simulink model "ThreePhaseVectorControl"  (R2020a)
settings: Solver=ode15s  StartTime=0.0  StopTime=2.5  MaxStep=1e-6  RelTol=1e-6
model workspace (MAT data in the model file):
  frequency = 1
values from neighbouring files (symbols this model uses):
  Buffer = 500    [PLLFYP.m]
  Ki_PLL = 0.005    [PLLFYP.m]
  Kp_PLL = 0.05    [PLLFYP.m]
  Kp_VSC = 500    [PLLFYP.m]
  Lf = 0.005    [PLLFYP.m]
  Lg = XR*Rg/(100*pi)    [PLLFYP.m]
  MPM_Ts = 1/5000    (= 0.0002)    [PLLFYP.m]
  Rf = 0.1    [PLLFYP.m]
  Rg = sqrt((1/(1+XR^2))*((500^2)/(Pn*SCR))^2)    [PLLFYP.m]
  Vdc = 2000    [PLLFYP.m]
  wL = 2*pi*50*Lf    (= 1.57079632679)    [PLLFYP.m]
  wn = 3000    [PLLFYP.m]
  zeta = 0.707    [PLLFYP.m]
undefined symbols (not defined in the file or in its folder): Ki_PQ, Kp_PQ, mpm_wc, plecs, Q, Q_KF, R, wb, wc, wc1, wc2
libraries: powerlib_meascontrol x57, powerlib x25, simulink x4, eeStairGenerator x4, powerlib_extras x2, cstblocks x2
(part 1 of 4)
settings Model: SimulationMode=accelerator  Creator=behroozb  LastModifiedBy=aaron
settings SolverCC: MaxConsecutiveZCs=10000  ZeroCrossAlgorithm=Adaptive  AlgebraicLoopSolver=LineSearch
settings DataIOCC: ReturnWorkspaceOutputs=off
settings OptimizationCC: LifeSpan=inf
settings DebuggingCC: IgnoredZcDiagnostic=none  SFUnexpectedBacktrackingDiag=warning  SFNoUnconditionalDefaultTransitionDiag=warning  SFExecutionAtInitializationDiag=none  ArithmeticOperatorsInVariantConditions=warning
settings SFSimCC: SimUseLocalCustomCode=off  CustomCodeUndefinedFunction=UseInterfaceOnly
settings RTWCC: RTWUseLocalCustomCode=off
settings CodeAppCC: StateflowObjectComments=on
settings GRTTargetCC: TargetLangStandard=C89/C90 (ANSI)
settings ConfigComp: CovMetricSettings=dw  CovHtmlReporting=on  CovSaveCumulativeToWorkspaceVar=on  CovSaveSingleToWorkspaceVar=on  CovExternalEMLEnable=off
settings SimscapeCC: SimscapeNormalizeSystem=off

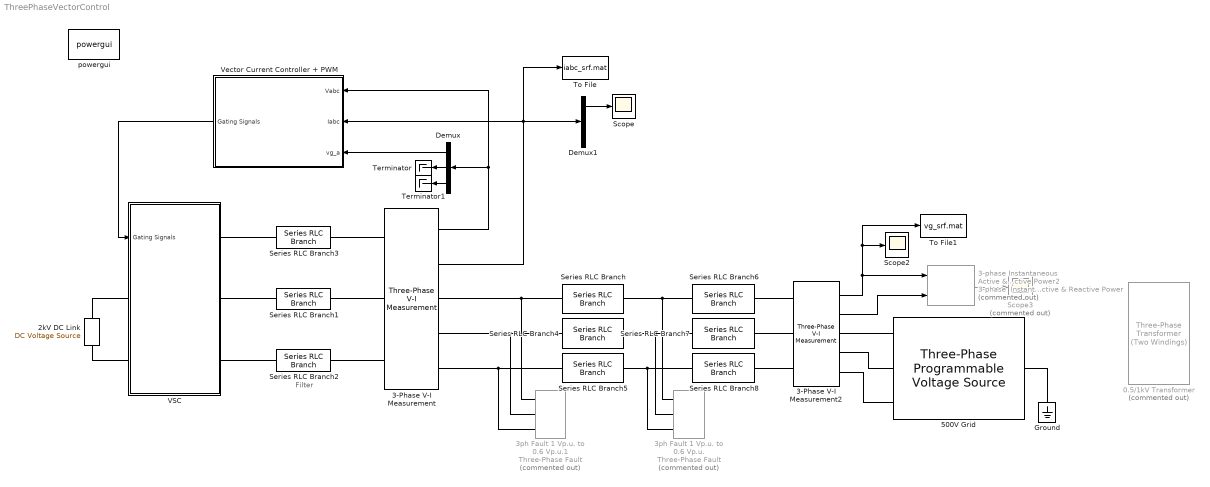
== system ThreePhaseVectorControl ==
  note: Filter
  0.5/1kV Transformer : powerlib/Elements/Three-Phase Transformer (Two Windings)  Commented=on  Winding1Connection=Yg  Winding2Connection=Yg  CoreType=Three single-phase transformers  SetSaturation=off  Hysteresis=off  DataFile='hysteresis'  SetInitialFlux=off  Measurements=None  UNITS=pu  NominalPower=[1e5 , 50]  Winding1=[500 , 0 , 0]  Winding2=[1000 , 0 , 0]  Rm=1e6  Lm=inf  L0=0.5  Saturation=[0 0;2.2531e-05 1065.2;0.0093878 1349.3]  InitialFluxes=[ 0.8 , -0.8 , 0.7 ]  BreakLoop=off  DiscreteSolver=Trapezoidal iterative  DataType=off  TransfoNumber=1
  2kV DC Link : powerlib/Electrical Sources/DC Voltage Source  Amplitude=Vdc  Measurements=None
  3-Phase V-I Measurement : powerlib/Measurements/Three-Phase V-I Measurement  VoltageMeasurement=phase-to-ground  SetLabelV=off  LabelV=Vabc  Vpu=off  VpuLL=off  CurrentMeasurement=yes  SetLabelI=off  LabelI=Iabc  Ipu=off  Pbase=100e6  Vbase=500e3  OutputType=Complex  PhasorSimulation=off  PSBequivalent=0
  3-Phase V-I Measurement2 : powerlib/Measurements/Three-Phase V-I Measurement  VoltageMeasurement=phase-to-ground  SetLabelV=off  LabelV=Vabc  Vpu=off  VpuLL=off  CurrentMeasurement=yes  SetLabelI=off  LabelI=Iabc  Ipu=off  Pbase=100e6  Vbase=500e3  OutputType=Complex  PhasorSimulation=off  PSBequivalent=0
  3-phase Instantaneous Active & Reactive Power2 : powerlib_extras/Measurements/3-phase  Instantaneous  Active & Reactive Power  Commented=on
      settings: SourceProductBaseCode=PS
  3ph Fault 1 Vp.u. to 0.6 Vp.u. : powerlib/Elements/Three-Phase Fault  Commented=on  InitialStates=0  FaultA=on  FaultB=on  FaultC=on  GroundFault=on  SwitchTimes=[0.35 0.43]  External=off  SwitchStatus=NaN  FaultResistance=9.2  GroundResistance=0.0001  SnubberResistance=inf  SnubberCapacitance=inf  Measurements=None
  3ph Fault 1 Vp.u. to 0.6 Vp.u.1 : powerlib/Elements/Three-Phase Fault  Commented=on  InitialStates=0  FaultA=on  FaultB=on  FaultC=on  GroundFault=on  SwitchTimes=[0.35 0.43]  External=off  SwitchStatus=NaN  FaultResistance=9.2  GroundResistance=0.0001  SnubberResistance=inf  SnubberCapacitance=inf  Measurements=None
  500V Grid : powerlib/Electrical Sources/Three-Phase Programmable Voltage Source  PositiveSequence=[500 0 50]  VariationEntity=None  VariationType=Step  VariationTypeAlt=Ramp  VariationStep=-0.1  VariationRate=-1  VariationMagnitude=0.1  VariationFrequency=1  VariationTiming=[0.4 0.5]  VariationPhaseA=off  Amplitudes=[1 0.8 1.2 1.0]  TimeValues=[0 0.1 0.15 0.2]  HarmonicGeneration=off  HarmonicA=[1 0.2 -25 2]  HarmonicB=[2 0.0 35 2]  Timing="[0.05  3]"  BusType=swing  Pref=0  Qref=0  Qmin=-inf  Qmax=inf
  Demux : Demux  Outputs=3
  Demux1 : Demux  Outputs=3
  Ground : powerlib/Elements/Ground  LConnTagsString=a
  Scope : Scope
  Scope2 : Scope
  Scope3 : Scope  Commented=on
  Series RLC Branch{,4..8} (6 alike) : powerlib/Elements/Series RLC Branch  LConnTagsString=__new0  RConnTagsString=__new0  BranchType=RL  Resistance=Rg/2  Inductance=Lg/2  SetiL0=off  InitialCurrent=0  Capacitance=1e-6  Setx0=off  InitialVoltage=0  Measurements=None
  Series RLC Branch1 : powerlib/Elements/Series RLC Branch  LConnTagsString=__new0  RConnTagsString=__new0  BranchType=RL  Resistance=Rf  Inductance=Lf  SetiL0=off  InitialCurrent=0  Capacitance=1.0  Setx0=off  InitialVoltage=0  Measurements=None
  Series RLC Branch2 : powerlib/Elements/Series RLC Branch  LConnTagsString=__new0  RConnTagsString=__new0  BranchType=RL  Resistance=Rf  Inductance=Lf  SetiL0=off  InitialCurrent=0  Capacitance=1.0  Setx0=off  InitialVoltage=0  Measurements=None
  Series RLC Branch3 : powerlib/Elements/Series RLC Branch  LConnTagsString=__new0  RConnTagsString=__new0  BranchType=RL  Resistance=Rf  Inductance=Lf  SetiL0=off  InitialCurrent=0  Capacitance=1.0  Setx0=off  InitialVoltage=0  Measurements=None
  Terminator : Terminator
  Terminator1 : Terminator
  To File : ToFile  Filename=iabc_srf.mat  SaveFormat=Timeseries
  To File1 : ToFile  Filename=vg_srf.mat  SaveFormat=Timeseries
  VSC : Subsystem
  Vector Current Controller + PWM : Subsystem
  powergui : powerlib/powergui  Priority=1  SimulationMode=Continuous  SampleTime=10e-6  frequency=60  Iterations=50  frequencyindice=50  Pbase=100e6  ErrMax=1e-4  UnitsV=kV  UnitsW=MW  buscounter=0  FunctionMessages=off  echomessages=off  EnableUseOfTLC=off  CurrentSourceSwitches=off  DisableSnubberDevices=off  DisableRonSwitches=off  DisableVfSwitches=off  DisplayEquations=off  AutomaticDiscreteSolvers=off  SolverType=Tustin/Backward Euler (TBE)  Interpol=off  ExternalGateDelay=off  methode=off  Ts=100  x0status=blocks  SPID=on  SwTol=0  HookPort=off  NonlinearTolerance=1e-4  nMaxIteration=100  ContinueOnMaxIteration=off  RestoreLinks=warning  ResistiveCurrentMeasurement=off  Frange=[0:2:500]  Ylog=off  Xlog=on  ShowGrid=off  save=off  variable=ZData  structure=ScopeData1  ZoomFFT=off  StartTime=0.4  cycles=20  DisplayStyle=1  fundamental=50  FreqAxis=off  MaxFrequency=150  frequencyindicesteady=1  RmsSteady=1  display=off
  wires:
  Vector Current Controller + PWM/1(Gating Signals) -> VSC/1(Gating Signals)
  3-Phase V-I Measurement/1 -> Vector Current Controller + PWM/1(Vabc), Demux/1
  Demux/1 -> Vector Current Controller + PWM/3(vg_a)
  Demux/2 -> Terminator/1
  Demux/3 -> Terminator1/1
  3-Phase V-I Measurement/2 -> Demux1/1, To File/1, Vector Current Controller + PWM/2(Iabc)
  Demux1/1 -> Scope/1
  3-Phase V-I Measurement2/2 -> 3-phase Instantaneous Active & Reactive Power2/2
  3-phase Instantaneous Active & Reactive Power2/1 -> Scope3/1
  3-Phase V-I Measurement2/1 -> 3-phase Instantaneous Active & Reactive Power2/1, To File1/1, Scope2/1
  connections:
  2kV DC Link/RConn1 -- VSC/LConn1
  2kV DC Link/LConn1 -- VSC/LConn2
  Series RLC Branch3/LConn1 -- VSC/RConn1
  Series RLC Branch1/LConn1 -- VSC/RConn2
  Series RLC Branch2/LConn1 -- VSC/RConn3
  500V Grid/LConn1 -- Ground/LConn1
  3-Phase V-I Measurement/LConn1 -- Series RLC Branch3/RConn1
  3-Phase V-I Measurement/LConn2 -- Series RLC Branch1/RConn1
  Series RLC Branch2/RConn1 -- 3-Phase V-I Measurement/LConn3
  Series RLC Branch6/LConn1 -- 3ph Fault 1 Vp.u. to 0.6 Vp.u./LConn1 -- Series RLC Branch/RConn1
  Series RLC Branch7/LConn1 -- 3ph Fault 1 Vp.u. to 0.6 Vp.u./LConn2 -- Series RLC Branch4/RConn1
  Series RLC Branch8/LConn1 -- 3ph Fault 1 Vp.u. to 0.6 Vp.u./LConn3 -- Series RLC Branch5/RConn1
  3-Phase V-I Measurement2/LConn1 -- Series RLC Branch6/RConn1
  3-Phase V-I Measurement2/LConn2 -- Series RLC Branch7/RConn1
  3-Phase V-I Measurement2/LConn3 -- Series RLC Branch8/RConn1
  3-Phase V-I Measurement2/RConn1 -- 500V Grid/RConn1
  3-Phase V-I Measurement2/RConn2 -- 500V Grid/RConn2
  3-Phase V-I Measurement2/RConn3 -- 500V Grid/RConn3
  3-Phase V-I Measurement/RConn1 -- 3ph Fault 1 Vp.u. to 0.6 Vp.u.1/LConn1 -- Series RLC Branch/LConn1
  Series RLC Branch4/LConn1 -- 3ph Fault 1 Vp.u. to 0.6 Vp.u.1/LConn2 -- 3-Phase V-I Measurement/RConn2
  3-Phase V-I Measurement/RConn3 -- 3ph Fault 1 Vp.u. to 0.6 Vp.u.1/LConn3 -- Series RLC Branch5/LConn1

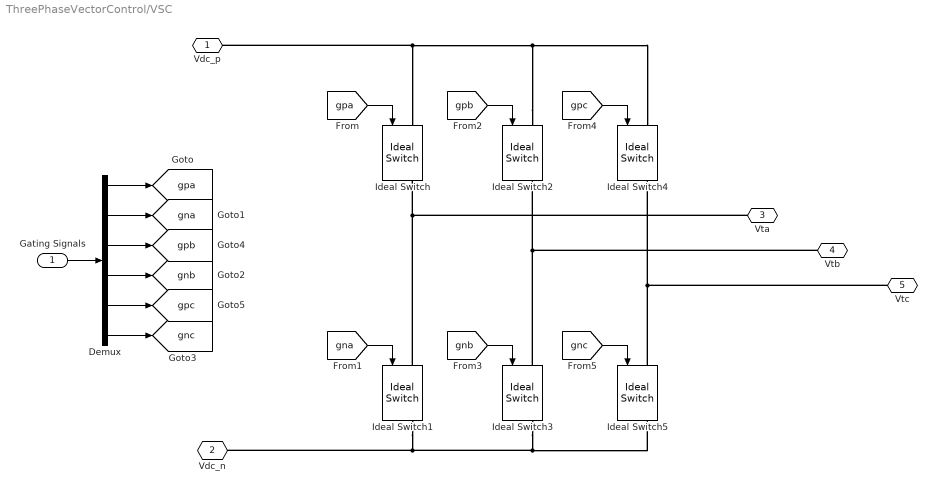
== system ThreePhaseVectorControl/VSC ==
  Gating Signals : Inport
  Demux : Demux  Outputs=6
  Ideal Switch{,1..5} (6 alike) : powerlib/Power Electronics/Ideal Switch  Ron=1e-6  Lon=0  IC=0  Rs=1e6  Cs=inf  Measurements=on
  Vdc_p : PMIOPort  Side=Left
  Vdc_n : PMIOPort  Port=2  Side=Left
  Vta : PMIOPort  Port=3  Side=Right
  Vtb : PMIOPort  Port=4  Side=Right
  Vtc : PMIOPort  Port=5  Side=Right
  tag scope: gna=global, gnb=global, gnc=global, gpa=global, gpb=global, gpc=global
  wires:
  [gpa] -> Ideal Switch/1
  [gpb] -> Ideal Switch2/1
  [gpc] -> Ideal Switch4/1
  [gna] -> Ideal Switch1/1
  [gnb] -> Ideal Switch3/1
  [gnc] -> Ideal Switch5/1
  Demux/3 -> [gpb]
  Demux/2 -> [gna]
  Demux/1 -> [gpa]
  Demux/4 -> [gnb]
  Demux/5 -> [gpc]
  Demux/6 -> [gnc]
  Gating Signals/1 -> Demux/1
  connections:
  Ideal Switch5/LConn1 -- Ideal Switch4/RConn1 -- Vtc/RConn1
  Ideal Switch3/LConn1 -- Ideal Switch2/RConn1 -- Vtb/RConn1
  Ideal Switch3/RConn1 -- Ideal Switch1/RConn1 -- Vdc_n/RConn1 -- Ideal Switch5/RConn1
  Ideal Switch1/LConn1 -- Vta/RConn1 -- Ideal Switch/RConn1
  Ideal Switch2/LConn1 -- Vdc_p/RConn1 -- Ideal Switch/LConn1 -- Ideal Switch4/LConn1

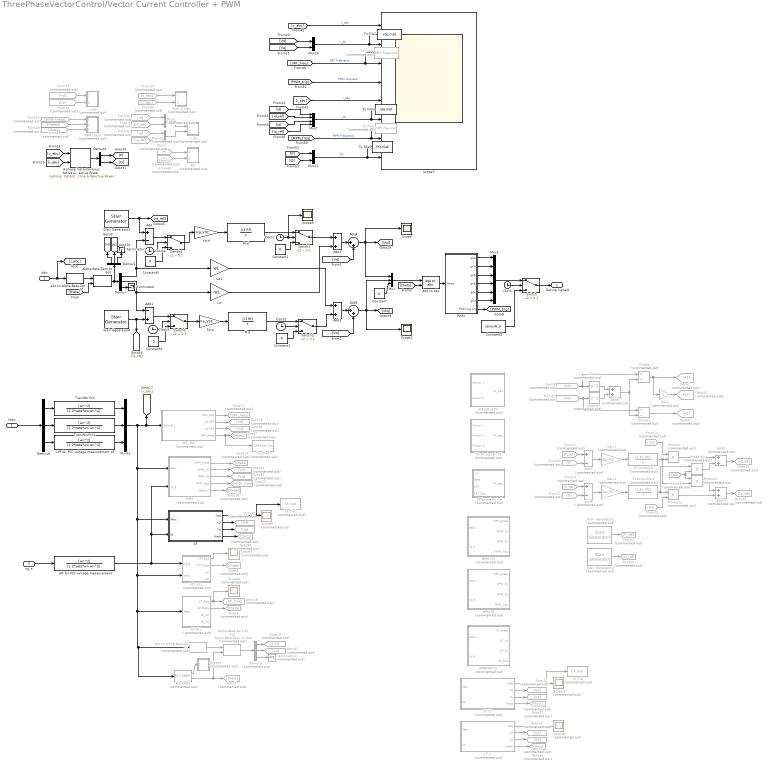
== system ThreePhaseVectorControl/Vector Current Controller + PWM ==
  Vabc : Inport
  Iabc : Inport  Port=2
  vg_a : Inport  Port=3
  3-phase Instantaneous Active & Reactive Power : powerlib_extras/Measurements/3-phase  Instantaneous  Active & Reactive Power
      settings: SourceProductBaseCode=PS
  Add : Sum  Inputs=+-
  Add1 : Sum  Inputs=-+
  Add10 : Sum  Commented=on
  Add2 : Sum
  Add3 : Sum
  Add4 : Sum  Inputs=|++
  Add5 : Sum  Inputs=|++
  Add6 : Sum  Commented=on
  Add7 : Sum  Commented=on  Inputs=+-
  Add8 : Sum  Commented=on  Inputs=+-
  Add9 : Sum  Commented=on
  Alpha-Beta-Zero to dq0 : powerlib_meascontrol/Transformations/Alpha-Beta-Zero to dq0  Alignment=Aligned with phase A axis
  Alpha-Beta-Zero to dq1 : powerlib_meascontrol/Transformations/Alpha-Beta-Zero to dq0  Commented=on  Alignment=Aligned with phase A axis
  CF : Subsystem
  CF (2) : Subsystem  Commented=on
  CF 2 : Subsystem  Commented=on
  CF based on i_d : Subsystem  Commented=on
  Clock{,1..4} (5 alike) : Clock
      settings: Decimation=100
  Constant{,1,3..5} (5 alike) : Constant  Value=0
  Constant2 : Constant  Value=zeros(6,1)
  Demux : Demux  Outputs=3
  Demux1 : Demux  Outputs=3
  Demux4 : Demux  Outputs=2
  Demux5 : Demux  Commented=on  Outputs=3
  Demux6 : Demux  Outputs=3
  Divide : Product  Commented=on  Inputs=*/
  Divide1 : Product  Commented=on  Inputs=*/
  FFT_PLL : Subsystem  Commented=on
  From10 : From  Commented=on  GotoTag=Vq
  From11 : From  Commented=on  GotoTag=P_ref
  From12 : From  Commented=on  GotoTag=Q
  From13 : From  Commented=on  GotoTag=Vd
  From14 : From  Commented=on  GotoTag=Vq
  From17 : From  Commented=on  GotoTag=MPM_theta
  From18 : From  Commented=on  GotoTag=theta0
  From19 : From  Commented=on  GotoTag=theta
  From22 : From  Commented=on  GotoTag=P
  From23 : From  Commented=on  GotoTag=Q_ref
  From24 : From  Commented=on  GotoTag=A1
  From25 : From  Commented=on  GotoTag=A3
  From26 : From  Commented=on  GotoTag=A2
  From34 : From  Commented=on  GotoTag=id
  From35 : From  Commented=on  GotoTag=iq
  From36 : From  Commented=on  GotoTag=i_abc
  From37 : From  Commented=on  GotoTag=v_abc
  From39 : From  Commented=on  GotoTag=P
  From40 : From  Commented=on  GotoTag=Q
  From7 : From  Commented=on  GotoTag=id_ref
  From8 : From  Commented=on  GotoTag=iq_ref
  From9 : From  Commented=on  GotoTag=Vd
  Gain : Gain  Commented=on  Gain=-1
  Gain1 : Gain  Commented=on  Gain=Kp_PQ
  Gain2 : Gain  Commented=on  Gain=Kp_PQ
  Goto1 : Goto  Commented=on  GotoTag=A1
  Goto11 : Goto  Commented=on  GotoTag=SRF_freq
  Goto12 : Goto  Commented=on  GotoTag=MPM_freq
  Goto{2,4..5,7,13,27,32,39} (8 alike) : Goto  Commented=on  GotoTag=theta
  Goto{14,19,25,33,35,37} (6 alike) : Goto  Commented=on  GotoTag=Vd
  Goto{15,26,34,36,38,47} (6 alike) : Goto  Commented=on  GotoTag=Vq
  Goto16 : Goto  Commented=on  GotoTag=KF_freq
  Goto18 : Goto  Commented=on  GotoTag=theta0
  Goto40 : Goto  Commented=on  GotoTag=A3
  Goto41 : Goto  Commented=on  GotoTag=id_ref
  Goto42 : Goto  Commented=on  GotoTag=iq_ref
  Goto43 : Goto  Commented=on  GotoTag=P_ref
  Goto44 : Goto  Commented=on  GotoTag=Q_ref
  Goto6 : Goto  Commented=on  GotoTag=A2
  KF_PLL : Subsystem  Commented=on
  Kp-d : Gain  Gain=Kp_VSC
  Kp-q : Gain  Gain=Kp_VSC
  LPF for PCC voltage measurement : TransferFcn  Numerator=[wn^2]  Denominator=[1 2*zeta*wn wn^2]
  LPF for PCC voltage measurement x3 : TransferFcn  Numerator=[wn^2]  Denominator=[1 2*zeta*wn wn^2]
  Lw : Gain  Gain=-wL
  Lw1 : Gain  Gain=wL
  MPM : Subsystem  Commented=on
  MPM CF : Subsystem  Commented=on
  MPM CF1 : Subsystem  Commented=on
  MPM theta : Subsystem  Commented=on  LoadFcn=plecs('sl', 300);  InitFcn=plecs('sl', 314);  StartFcn=plecs('sl', 308);  StopFcn=plecs('sl', 309);  mask{Settings=<binary blob, 1428 chars, not shown>}
      mask init:
      | plecs('sl', 315);
      settings: CopyFcn=plecs('sl', 303);  DeleteFcn=plecs('sl', 305);  UndoDeleteFcn=plecs('sl', 306);  PreSaveFcn=plecs('sl', 311);  NameChangeFcn=plecs('sl', 310);  DestroyFcn=plecs('sl', 307);  OpenFcn=plecs('sl', 302);  ErrorFcn=plerrorfcn
      mask Display: plot([0.1 0.9 0.9 0.1 0.1], [0.9 0.9 0.5 0.5 0.9])
  MPM/SRF CF : Subsystem  Commented=on
  Mux : Mux  Inputs=3
  Mux1 : Mux  Inputs=6
  Mux10 : Mux  Inputs=2
  Mux11 : Mux  Inputs=2
  Mux12 : Mux  Inputs=3
  Mux2 : Mux  Commented=on  Inputs=2
  Mux3 : Mux  Commented=on  Inputs=2
  Mux7 : Mux
  PI Controller : TransferFcn  Commented=on  Numerator=[1 Ki_PQ]  Denominator=[1 0]
  PI Controller1 : TransferFcn  Commented=on  Numerator=[1 Ki_PQ]  Denominator=[1 0]
  PI-d : TransferFcn  Numerator=[Lf Rf]  Denominator=[1 0]
  PI-q : TransferFcn  Numerator=[Lf Rf]  Denominator=[1 0]
  PLL (3ph) : powerlib_meascontrol/PLL/PLL (3ph)  Commented=on  Fmin=45  Par_Init=[0, 50]  ParK=[180, 3200, 1]  TcD=1e-4  MaxRateChangeFreq=12  FilterCutOffFreq=25  Ts=1e-4  AGC=on
  PQ : Subsystem  Commented=on  LoadFcn=plecs('sl', 300);  InitFcn=plecs('sl', 314);  StartFcn=plecs('sl', 308);  StopFcn=plecs('sl', 309);  mask{Settings=<binary blob, 1208 chars, not shown>}
      mask init:
      | plecs('sl', 315);
      settings: CopyFcn=plecs('sl', 303);  DeleteFcn=plecs('sl', 305);  UndoDeleteFcn=plecs('sl', 306);  PreSaveFcn=plecs('sl', 311);  NameChangeFcn=plecs('sl', 310);  DestroyFcn=plecs('sl', 307);  OpenFcn=plecs('sl', 302);  ErrorFcn=plerrorfcn
      mask Display: plot([0.1 0.9 0.9 0.1 0.1], [0.9 0.9 0.5 0.5 0.9])
  PWM : Subsystem
  Product{,1..3} (4 alike) : Product  Commented=on
  SRF_PLL : Subsystem  Commented=on
  Scope : Scope
  Scope1 : Subsystem  Commented=on  LoadFcn=plecs('sl', 300);  InitFcn=plecs('sl', 314);  StartFcn=plecs('sl', 308);  StopFcn=plecs('sl', 309);  mask{Settings=<binary blob, 1052 chars, not shown>}
      mask init:
      | plecs('sl', 315);
      settings: CopyFcn=plecs('sl', 303);  DeleteFcn=plecs('sl', 305);  UndoDeleteFcn=plecs('sl', 306);  PreSaveFcn=plecs('sl', 311);  NameChangeFcn=plecs('sl', 310);  DestroyFcn=plecs('sl', 307);  OpenFcn=plecs('sl', 302);  ErrorFcn=plerrorfcn
      mask Display: plot([0.1 0.9 0.9 0.1 0.1], [0.9 0.9 0.5 0.5 0.9])
  Scope2 : Scope
  Scope3 : Scope
  Scope{4..6,8..9} (5 alike) : Scope  Commented=on
  Scope7 : Scope  NumInputPorts=8
  Square : Math  Commented=on  Operator=square  SaturateOnIntegerOverflow=on
  Square1 : Math  Commented=on  Operator=square  SaturateOnIntegerOverflow=on
  Stair Generator1 : eeStairGenerator/Stair Generator  Commented=on  LabelModeActiveChoice=Discrete  TimeInput=[0 0.15]  AmplitudeInput=[0 1e4]  SampleTime=0.01  RepeatPattern=off  OutDataTypeStr=double
      settings: SourceProductBaseCode=PS
  Stair Generator2 : eeStairGenerator/Stair Generator  Commented=on  LabelModeActiveChoice=Discrete  TimeInput=[0]  AmplitudeInput=[0]  SampleTime=0.01  RepeatPattern=off  OutDataTypeStr=double
      settings: SourceProductBaseCode=PS
  Stair Generator3 : eeStairGenerator/Stair Generator  LabelModeActiveChoice=Discrete  TimeInput=[0 0.15]  AmplitudeInput=[0 50]  SampleTime=0.01  RepeatPattern=off  OutDataTypeStr=double
      settings: SourceProductBaseCode=PS
  Stair Generator4 : eeStairGenerator/Stair Generator  LabelModeActiveChoice=Discrete  TimeInput=[0]  AmplitudeInput=[0]  SampleTime=0.01  RepeatPattern=off  OutDataTypeStr=double
      settings: SourceProductBaseCode=PS
  Standard CF : Subsystem  Commented=on
  Switch{,1..4} (5 alike) : Switch  Criteria=u2 > Threshold  Threshold=0.1
  Terminator : Terminator
  Terminator1 : Terminator
  Terminator2 : Terminator  Commented=on
  Three signals CF : Subsystem  Commented=on
  To File : ToFile  Commented=on  Filename=CF.mat  SaveFormat=Timeseries
  To File1 : ToFile  Commented=on  Filename=CF.mat  SaveFormat=Timeseries
  To File2 : ToFile  Commented=on  Filename=MPM_freq.mat  SaveFormat=Timeseries
  To File3 : ToFile  Filename=idq.mat  SaveFormat=Timeseries
  To File4 : ToFile  Commented=on  Filename=SRF_freq.mat  SaveFormat=Timeseries
  To File5 : ToFile  Filename=PQ.mat  SaveFormat=Timeseries
  To File6 : ToFile  Commented=on  Filename=SRFtheta.mat  SaveFormat=Timeseries
  To File7 : ToFile  Filename=vdq.mat  SaveFormat=Timeseries
  Transfer Fcn : TransferFcn  Numerator=[wn^2]  Denominator=[1 2*zeta*wn wn^2]
  Transfer Fcn1 : TransferFcn  Numerator=[wn^2]  Denominator=[1 2*zeta*wn wn^2]
  Vabc & Iabc : Subsystem  Commented=on  LoadFcn=plecs('sl', 300);  InitFcn=plecs('sl', 314);  StartFcn=plecs('sl', 308);  StopFcn=plecs('sl', 309);  mask{Settings=<binary blob, 1272 chars, not shown>}
      mask init:
      | plecs('sl', 315);
      settings: CopyFcn=plecs('sl', 303);  DeleteFcn=plecs('sl', 305);  UndoDeleteFcn=plecs('sl', 306);  PreSaveFcn=plecs('sl', 311);  NameChangeFcn=plecs('sl', 310);  DestroyFcn=plecs('sl', 307);  OpenFcn=plecs('sl', 302);  ErrorFcn=plerrorfcn
      mask Display: plot([0.1 0.9 0.9 0.1 0.1], [0.9 0.9 0.5 0.5 0.9])
  abc to Alpha-Beta-Zero1 : powerlib_meascontrol/Transformations/abc to Alpha-Beta-Zero
  abc to Alpha-Beta-Zero2 : powerlib_meascontrol/Transformations/abc to Alpha-Beta-Zero  Commented=on
  dq0 to abc : powerlib_meascontrol/Transformations/dq0 to abc  Alignment=Aligned with phase A axis
  i_dq : Subsystem  Commented=on  LoadFcn=plecs('sl', 300);  InitFcn=plecs('sl', 314);  StartFcn=plecs('sl', 308);  StopFcn=plecs('sl', 309);  mask{Settings=<binary blob, 1256 chars, not shown>}
      mask init:
      | plecs('sl', 315);
      settings: CopyFcn=plecs('sl', 303);  DeleteFcn=plecs('sl', 305);  UndoDeleteFcn=plecs('sl', 306);  PreSaveFcn=plecs('sl', 311);  NameChangeFcn=plecs('sl', 310);  DestroyFcn=plecs('sl', 307);  OpenFcn=plecs('sl', 302);  ErrorFcn=plerrorfcn
      mask Display: plot([0.1 0.9 0.9 0.1 0.1], [0.9 0.9 0.5 0.5 0.9])
  v_dq : Subsystem  Commented=on  LoadFcn=plecs('sl', 300);  InitFcn=plecs('sl', 314);  StartFcn=plecs('sl', 308);  StopFcn=plecs('sl', 309);  mask{Settings=<binary blob, 1220 chars, not shown>}
      mask init:
      | plecs('sl', 315);
      settings: CopyFcn=plecs('sl', 303);  DeleteFcn=plecs('sl', 305);  UndoDeleteFcn=plecs('sl', 306);  PreSaveFcn=plecs('sl', 311);  NameChangeFcn=plecs('sl', 310);  DestroyFcn=plecs('sl', 307);  OpenFcn=plecs('sl', 302);  ErrorFcn=plerrorfcn
      mask Display: plot([0.1 0.9 0.9 0.1 0.1], [0.9 0.9 0.5 0.5 0.9])
  Gating Signals : Outport  VectorParamsAs1DForOutWhenUnconnected=off
  wires:
  Iabc/1 -> [i_abc], abc to Alpha-Beta-Zero1/1
  abc to Alpha-Beta-Zero1/1 -> Alpha-Beta-Zero to dq0/1
  [theta] -> Alpha-Beta-Zero to dq0/2
  Alpha-Beta-Zero to dq0/1 -> Demux1/1, Demux/1
  Demux/2 -> Lw/1, Add1/1
  Demux/1 -> Add/2, Lw1/1
  Add2/1 -> Add4/1
  Add3/1 -> Add5/1
  [theta] -> dq0 to abc/2
  dq0 to abc/1 -> PWM/1(Vtabc)
  Constant/1 -> Mux/3
  Mux/1 -> dq0 to abc/1
  [Vd] -> Add4/2
  [Vq] -> Add5/2
  Lw1/1 -> Add3/1
  Lw/1 -> Add2/2
  Kp-d/1 -> PI-d/1
  Kp-q/1 -> PI-q/1
  Demux/3 -> Terminator/1
  PWM/1(gpa) -> Mux1/1
  PWM/2(gna) -> Mux1/2
  PWM/3(gpb) -> Mux1/3
  PWM/4(gnb) -> Mux1/4
  PWM/5(gpc) -> Mux1/5
  PWM/6(gnc) -> Mux1/6
  Switch/1 -> Gating Signals/1
  Clock/1 -> Switch/2
  Clock1/1 -> Scope3/1, Switch1/2
  Switch1/1 -> Add2/1
  Clock2/1 -> Switch2/2
  Switch2/1 -> Add3/2
  PI-d/1 -> Switch1/1
  Constant1/1 -> Switch1/3
  PI-q/1 -> Switch2/1
  Constant3/1 -> Switch2/3
  Mux1/1 -> Switch/1
  Constant2/1 -> Switch/3
  Demux1/1 -> [id]
  Demux1/2 -> [iq]
  Demux1/3 -> Terminator1/1
  KF_PLL/2(KF_theta) -> Goto5/1
  FFT_PLL/2(FFT theta) -> Goto4/1
  FFT_PLL/1(FFT freq) -> Scope5/1
  KF_PLL/1(KF_freq) -> Scope4/1, Goto16/1
  From7/1 -> Mux2/2
  From8/1 -> Mux3/2
  3-phase Instantaneous Active & Reactive Power/1 -> Demux4/1
  [v_abc] -> 3-phase Instantaneous Active & Reactive Power/1
  [i_abc] -> 3-phase Instantaneous Active & Reactive Power/2
  From17/1 -> MPM theta/1(1)
  From18/1 -> MPM theta/2(2)
  From19/1 -> MPM theta/3(3)
  Mux2/1 -> i_dq/1(1)
  Mux3/1 -> i_dq/2(2)
  From34/1 -> Mux2/1
  From35/1 -> Mux3/1
  From37/1 -> Vabc & Iabc/1(1)
  From36/1 -> Vabc & Iabc/2(2)
  From14/1 -> v_dq/2(2)
  From13/1 -> v_dq/1(1)
  From40/1 -> PQ/2(2)
  From39/1 -> PQ/1(1)
  PLL (3ph)/1 -> Scope1/1(1)
  abc to Alpha-Beta-Zero2/1 -> Alpha-Beta-Zero to dq1/1
  Demux5/3 -> Terminator2/1
  Alpha-Beta-Zero to dq1/1 -> Demux5/1
  PLL (3ph)/2 -> Goto2/1, Alpha-Beta-Zero to dq1/2
  SRF_PLL/4(SRF_theta) -> To File6/1, Goto7/1
  PWM/7(PWM trig sin) -> [PWM_trig]
  Demux4/1 -> [P]
  Demux4/2 -> [Q]
  SRF_PLL/1(SRF_freq) -> Goto11/1
  [v_abc] -> Scope7/1  "v_abc"
  [SRF_freq] -> To File4/1, Scope7/3  "SRF Frequency"
  [PWM_trig] -> Scope7/4  "PWM compare"
  [MPM_freq] -> To File2/1, Scope7/7  "MPM Frequency"
  Mux10/1 -> To File7/1, Scope7/2  "v_dq"
  Mux11/1 -> To File5/1, Scope7/8  "PQ"
  Mux7/1 -> To File3/1, Scope7/6  "i_dq"
  [id_ref] -> Mux7/2
  [Vd] -> Mux10/1
  [i_abc] -> Scope7/5  "i_abc"
  [iq] -> Mux7/3
  [Vq] -> Mux10/2
  [id] -> Mux7/1
  [P] -> Mux11/1
  [iq_ref] -> Mux7/4
  [Q] -> Mux11/2
  Vabc/1 -> Demux6/1
  Mux12/1 -> [v_abc], SRF_PLL/1(Vabc-PLL), MPM/1(Vabc), FFT_PLL/2(Vabc), PLL (3ph)/1, abc to Alpha-Beta-Zero2/1, KF_PLL/1(Vabc), CF/1(Vabc)
  LPF for PCC voltage measurement/1 -> FFT_PLL/1(vg_a), MPM/2(vg_a), CF/2(Va)
  vg_a/1 -> LPF for PCC voltage measurement/1
  Add5/1 -> Scope2/1, Mux/2, [Vtq]
  Add4/1 -> Mux/1, [Vtd], Scope/1
  Demux6/1 -> Transfer Fcn/1
  Demux6/2 -> Transfer Fcn1/1
  Demux6/3 -> LPF for PCC voltage measurement x3/1
  Transfer Fcn/1 -> Mux12/1
  Transfer Fcn1/1 -> Mux12/2
  LPF for PCC voltage measurement x3/1 -> Mux12/3
  MPM/5(theta_0) -> Goto18/1
  MPM/4(MPM_freq) -> Goto12/1
  MPM/1(MPM_theta) -> Goto13/1
  CF 2/3(Vq) -> Goto15/1
  CF 2/2(Vd) -> Goto14/1
  CF 2/4(theta) -> Goto32/1
  CF 2/1(freq) -> Scope8/1
  MPM/3(MPM_Vq) -> Goto34/1
  MPM/2(MPM_Vd) -> Goto33/1
  SRF_PLL/3(Vq SRF) -> Goto36/1
  SRF_PLL/2(Vd SRF) -> Goto35/1
  CF/2(Vd) -> Goto37/1
  CF/4(theta) -> Goto39/1
  CF/1(freq) -> To File1/1, Scope6/1
  CF/3(Vq) -> Goto38/1
  CF (2)/2(Vd) -> Goto25/1
  CF (2)/3(Vq) -> Goto26/1
  CF (2)/1(freq) -> To File/1, Scope9/1
  CF (2)/4(theta) -> Goto27/1
  From9/1 -> Divide/1, Square/1
  From10/1 -> Divide1/1, Square1/1
  Square/1 -> Add6/1
  Square1/1 -> Add6/2
  Add6/1 -> Divide1/2, Divide/2
  Divide/1 -> Gain/1, Goto1/1
  Divide1/1 -> Goto6/1
  Gain/1 -> Goto40/1
  From11/1 -> Add7/1
  From22/1 -> Add7/2
  From12/1 -> Add8/2
  From23/1 -> Add8/1
  Gain1/1 -> PI Controller/1
  Add7/1 -> Gain1/1
  Gain2/1 -> PI Controller1/1
  Add8/1 -> Gain2/1
  PI Controller/1 -> Product3/2, Product/2
  From24/1 -> Product/1
  Product/1 -> Add9/1
  PI Controller1/1 -> Product1/1, Product2/1
  From25/1 -> Product1/2
  Product1/1 -> Add10/2
  Product2/1 -> Add9/2
  Product3/1 -> Add10/1
  From26/1 -> Product2/2, Product3/1
  Stair Generator1/1 -> Goto43/1
  Stair Generator2/1 -> Goto44/1
  Clock3/1 -> Switch3/2
  Constant4/1 -> Switch3/3
  Add1/1 -> Switch3/1
  Switch3/1 -> Kp-q/1
  Constant5/1 -> Switch4/3
  Clock4/1 -> Switch4/2
  Add/1 -> Switch4/1
  Switch4/1 -> Kp-d/1
  Add9/1 -> Goto41/1
  Add10/1 -> Goto42/1
  Stair Generator3/1 -> Add/1, [id_ref]
  Stair Generator4/1 -> Add1/2, [iq_ref]
  Demux5/1 -> Goto19/1
  Demux5/2 -> Goto47/1

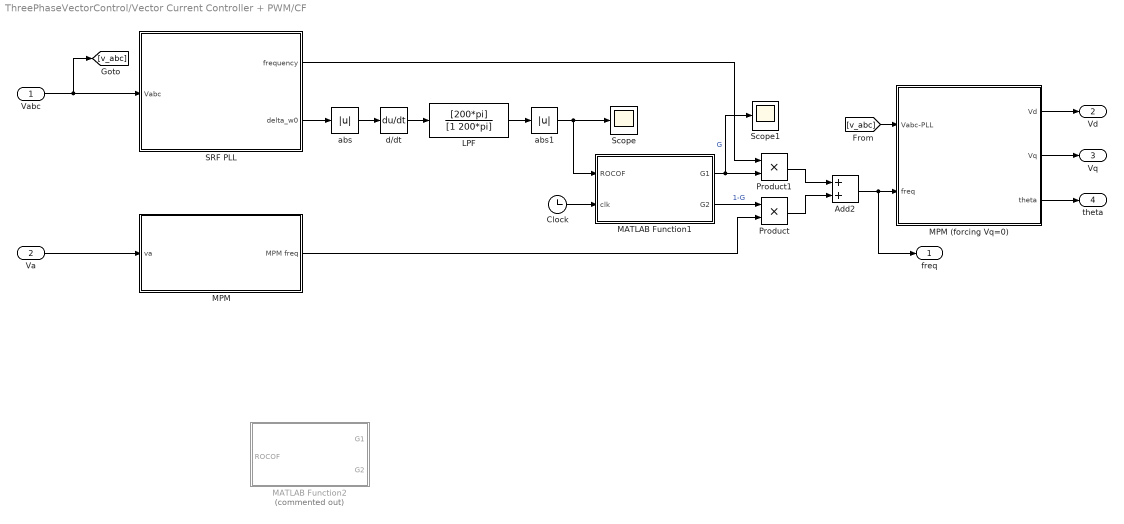
== system ThreePhaseVectorControl/Vector Current Controller + PWM/CF ==
  Vabc : Inport
  Va : Inport  Port=2
  Add2 : Sum
  Clock : Clock
  LPF : TransferFcn  Numerator=[200*pi]  Denominator=[1 200*pi]
  MATLAB Function1 : MATLAB Function  TreatAsAtomicUnit=on
  MATLAB Function2 : MATLAB Function  Commented=on  TreatAsAtomicUnit=on
  MPM : Subsystem
  MPM (forcing Vq=0) : Subsystem
  Product : Product
  Product1 : Product
  SRF PLL : Subsystem
  Scope : Scope
  Scope1 : Scope
  abs : Abs
  abs1 : Abs
  d/dt : Derivative
  freq : Outport
  Vd : Outport  Port=2  VectorParamsAs1DForOutWhenUnconnected=off
  Vq : Outport  Port=3  VectorParamsAs1DForOutWhenUnconnected=off
  theta : Outport  Port=4
  wires:
  Va/1 -> MPM/1(va)
  Product1/1 -> Add2/1
  Product/1 -> Add2/2
  SRF PLL/2(delta_w0) -> abs/1
  abs/1 -> d/dt/1
  d/dt/1 -> LPF/1
  MATLAB Function1/1(G1) -> Scope1/1, Product1/2  "G"
  MATLAB Function1/2(G2) -> Product/1  "1-G"
  SRF PLL/1(frequency) -> Product1/1
  MPM/1(MPM freq) -> Product/2
  Add2/1 -> freq/1, MPM (forcing Vq=0)/2(freq)
  MPM (forcing Vq=0)/1(Vd) -> Vd/1
  MPM (forcing Vq=0)/2(Vq) -> Vq/1
  MPM (forcing Vq=0)/3(theta) -> theta/1
  Vabc/1 -> [v_abc], SRF PLL/1(Vabc)
  [v_abc] -> MPM (forcing Vq=0)/1(Vabc-PLL)
  Clock/1 -> MATLAB Function1/2(clk)
  LPF/1 -> abs1/1
  abs1/1 -> MATLAB Function1/1(ROCOF), Scope/1

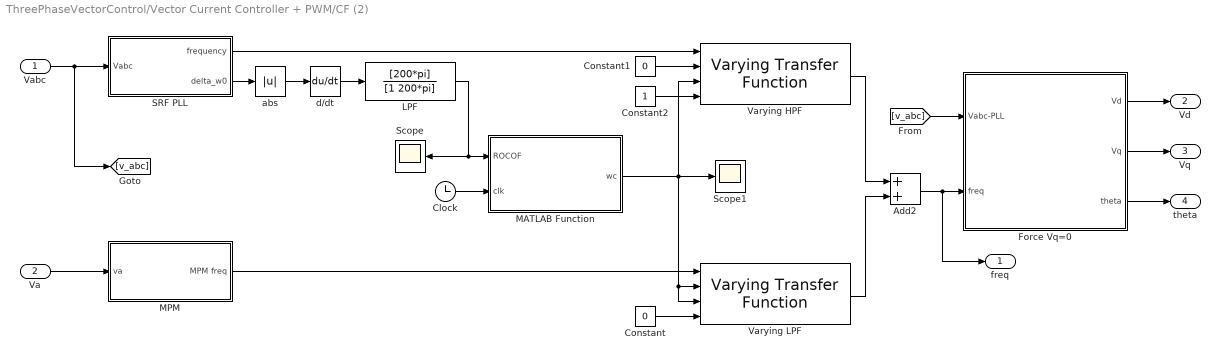
== system ThreePhaseVectorControl/Vector Current Controller + PWM/CF (2) ==
  Vabc : Inport
  Va : Inport  Port=2
  Add2 : Sum
  Clock : Clock
  Constant : Constant  Value=0
  Constant1 : Constant  Value=0
  Constant2 : Constant
  Force Vq=0 : Subsystem
  LPF : TransferFcn  Numerator=[200*pi]  Denominator=[1 200*pi]
  MATLAB Function : MATLAB Function  TreatAsAtomicUnit=on
  MPM : Subsystem
  SRF PLL : Subsystem
  Scope : Scope
  Scope1 : Scope
  Varying HPF : cstblocks/Linear Parameter Varying/Varying Transfer Function  N=1
  Varying LPF : cstblocks/Linear Parameter Varying/Varying Transfer Function  N=1
  abs : Abs
  d/dt : Derivative
  freq : Outport
  Vd : Outport  Port=2  VectorParamsAs1DForOutWhenUnconnected=off
  Vq : Outport  Port=3  VectorParamsAs1DForOutWhenUnconnected=off
  theta : Outport  Port=4
  wires:
  Va/1 -> MPM/1(va)
  SRF PLL/2(delta_w0) -> abs/1
  abs/1 -> d/dt/1
  d/dt/1 -> LPF/1
  LPF/1 -> Scope/1, MATLAB Function/1(ROCOF)
  Add2/1 -> freq/1, Force Vq=0/2(freq)
  Force Vq=0/1(Vd) -> Vd/1
  Force Vq=0/2(Vq) -> Vq/1
  Force Vq=0/3(theta) -> theta/1
  Vabc/1 -> SRF PLL/1(Vabc), [v_abc]
  [v_abc] -> Force Vq=0/1(Vabc-PLL)
  Constant/1 -> Varying LPF/4
  Varying LPF/1 -> Add2/2
  MPM/1(MPM freq) -> Varying LPF/1
  SRF PLL/1(frequency) -> Varying HPF/1
  Varying HPF/1 -> Add2/1
  Constant1/1 -> Varying HPF/2
  Constant2/1 -> Varying HPF/4
  MATLAB Function/1(wc) -> Varying LPF/3, Varying LPF/2, Scope1/1, Varying HPF/3
  Clock/1 -> MATLAB Function/2(clk)

== system ThreePhaseVectorControl/Vector Current Controller + PWM/CF 2 ==
  Vabc : Inport
  Va : Inport  Port=2
  Add2 : Sum
  LPF : TransferFcn  Numerator=[200*pi]  Denominator=[1 200*pi]
  MATLAB Function : MATLAB Function  TreatAsAtomicUnit=on
  MPM : Subsystem
  MPM (forcing Vq=0) : Subsystem
  Product : Product
  Product1 : Product
  SRF PLL : Subsystem
  abs : Abs
  d/dt : Derivative
  freq : Outport
  Vd : Outport  Port=2  VectorParamsAs1DForOutWhenUnconnected=off
  Vq : Outport  Port=3  VectorParamsAs1DForOutWhenUnconnected=off
  theta : Outport  Port=4
  wires:
  Va/1 -> MPM/1(va)
  MPM/1(MPM freq) -> MPM (forcing Vq=0)/2(MPM theta)
  Vabc/1 -> MPM (forcing Vq=0)/1(Vabc-PLL), SRF PLL/1(abc)
  Product1/1 -> Add2/1
  Product/1 -> Add2/2
  MPM (forcing Vq=0)/1(MPM_theta) -> Product/2
  SRF PLL/1(Vd) -> Vd/1
  SRF PLL/4(frequency) -> freq/1
  SRF PLL/2(Vq) -> Vq/1
  SRF PLL/3(delta_w0) -> abs/1
  abs/1 -> d/dt/1
  d/dt/1 -> LPF/1
  MATLAB Function/1(G1) -> Product1/2  "G"
  MATLAB Function/2(G2) -> Product/1  "1-G"
  LPF/1 -> MATLAB Function/1(ROCOF)
  Add2/1 -> theta/1, SRF PLL/2(wt)
  SRF PLL/5(theta) -> Product1/1

== system ThreePhaseVectorControl/Vector Current Controller + PWM/CF based on i_d ==
  i_d : Inport
  MPM : Inport  Port=2
  SRF : Inport  Port=3
  FFT_freq : Inport  Port=4
  CF : TransferFcn  Commented=on  Denominator=[1/50 1]
  CF_func : MATLAB Function  Commented=on  TreatAsAtomicUnit=on
  CF_freq : Outport
  wires:
  i_d/1 -> CF_func/1(i_d)
  SRF/1 -> CF_func/3(SRF)
  CF_func/1(CF_freq) -> CF/1
  FFT_freq/1 -> CF_func/4(FFT_freq)
  MPM/1 -> CF_func/2(MPM)
  CF/1 -> CF_freq/1

== system ThreePhaseVectorControl/Vector Current Controller + PWM/FFT_PLL ==
  vg_a : Inport
  Vabc : Inport  Port=2
  2*pi : Step  Time=0  After=2*pi  SampleTime=0
  Buffer : Buffer  N=3000  V=2999  ic=zeros(3000,1)  OutputFrames=off
  Clock3 : Clock
      settings: Decimation=100
  Constant1 : Constant  Value=1/50000
  Constant4 : Constant  Value=50
  Constant7 : Constant  Value=2*pi
  FFT PLL : MATLAB Function  TreatAsAtomicUnit=on
  Integrator2 : Integrator  UpperSaturationLimit=2*pi  LowerSaturationLimit=0  IgnoreLimit=on
  MPM (forcing Vq=0) : Subsystem
  Math Function2 : Math  Operator=mod  SignedPower=on  SaturateOnIntegerOverflow=on
  Product2 : Product  RndMeth=Zero
  Switch3 : Switch  Criteria=u2 > Threshold  Threshold=0.12
  Zero-Order Hold : ZeroOrderHold  SampleTime=1/50000
  FFT freq : Outport
  FFT theta : Outport  Port=2
  Vd : Outport  Port=3
  Vq : Outport  Port=4
  wires:
  Buffer/1 -> FFT PLL/1(data)
  Zero-Order Hold/1 -> Buffer/1
  vg_a/1 -> Zero-Order Hold/1
  Product2/1 -> Integrator2/1
  Integrator2/1 -> Math Function2/1
  2*pi/1 -> Product2/2
  Constant7/1 -> Math Function2/2
  Math Function2/1 -> MPM (forcing Vq=0)/2(FFT theta)
  MPM (forcing Vq=0)/1(FFT_theta) -> FFT theta/1
  MPM (forcing Vq=0)/2(Vd FFT) -> Vd/1
  MPM (forcing Vq=0)/3(Vq FFT) -> Vq/1
  Vabc/1 -> MPM (forcing Vq=0)/1(Vabc-PLL)
  Constant4/1 -> Switch3/3
  Clock3/1 -> Switch3/2
  FFT PLL/1(f) -> Switch3/1
  Switch3/1 -> FFT freq/1, Product2/1
  Constant1/1 -> FFT PLL/2(T)

== system ThreePhaseVectorControl/Vector Current Controller + PWM/KF_PLL ==
  Vabc : Inport
  KF/GAM : Subsystem
  Kalman Filter-based PLL : Subsystem
  MPM (forcing Vq=0) : Subsystem
  KF_freq : Outport
  KF_theta : Outport  Port=2
  KF_Vd : Outport  Port=3
  KF_Vq : Outport  Port=4
  wires:
  KF/GAM/1(KF_f) -> KF_freq/1
  MPM (forcing Vq=0)/1(KF_theta) -> KF_theta/1
  KF/GAM/2(KF theta) -> MPM (forcing Vq=0)/2(KF theta)
  MPM (forcing Vq=0)/2(Vd KF) -> KF_Vd/1
  MPM (forcing Vq=0)/3(Vq KF) -> KF_Vq/1
  Vabc/1 -> MPM (forcing Vq=0)/1(Vabc-PLL), KF/GAM/1(Vabc)

== system ThreePhaseVectorControl/Vector Current Controller + PWM/MPM ==
  Vabc : Inport
  vg_a : Inport  Port=2
  MPM : Subsystem
  MPM (forcing Vq=0) : Subsystem
  MPM_theta : Outport
  MPM_Vd : Outport  Port=2
  MPM_Vq : Outport  Port=3
  MPM_freq : Outport  Port=4
  theta_0 : Outport  Port=5
  wires:
  vg_a/1 -> MPM/1(va)
  MPM/1(freq) -> MPM_freq/1
  MPM (forcing Vq=0)/4(theta_0) -> theta_0/1
  MPM (forcing Vq=0)/1(MPM_theta) -> MPM_theta/1
  Vabc/1 -> MPM (forcing Vq=0)/1(Vabc-PLL)
  MPM (forcing Vq=0)/2(Vd MPM) -> MPM_Vd/1
  MPM (forcing Vq=0)/3(Vq MPM) -> MPM_Vq/1
  MPM/2(MPM theta) -> MPM (forcing Vq=0)/2(MPM theta)

== system ThreePhaseVectorControl/Vector Current Controller + PWM/MPM CF ==
  Vabc : Inport
  vg_a : Inport  Port=2
  MPM : Subsystem
  MPM (forcing Vq=0) : Subsystem
  MPM_theta : Outport
  MPM_Vd : Outport  Port=2
  MPM_Vq : Outport  Port=3
  MPM_freq : Outport  Port=4
  wires:
  vg_a/1 -> MPM/1(In1)
  MPM/1(Out1) -> MPM_freq/1
  MPM (forcing Vq=0)/1(MPM_theta) -> MPM_theta/1
  MPM/2(MPM theta) -> MPM (forcing Vq=0)/2(MPM theta)
  Vabc/1 -> MPM (forcing Vq=0)/1(Vabc-PLL)
  MPM (forcing Vq=0)/2(Vd MPM) -> MPM_Vd/1
  MPM (forcing Vq=0)/3(Vq MPM) -> MPM_Vq/1

== system ThreePhaseVectorControl/Vector Current Controller + PWM/MPM CF1 ==
  Vabc : Inport
  vg_a : Inport  Port=2
  MPM : Subsystem
  MPM (forcing Vq=0) : Subsystem
  MPM_theta : Outport
  MPM_Vd : Outport  Port=2
  MPM_Vq : Outport  Port=3
  MPM_freq : Outport  Port=4
  wires:
  vg_a/1 -> MPM/1(In1)
  MPM/1(Out1) -> MPM_freq/1
  MPM (forcing Vq=0)/1(MPM_theta) -> MPM_theta/1
  MPM/2(MPM theta) -> MPM (forcing Vq=0)/2(MPM theta)
  Vabc/1 -> MPM (forcing Vq=0)/1(Vabc-PLL)
  MPM (forcing Vq=0)/2(Vd MPM) -> MPM_Vd/1
  MPM (forcing Vq=0)/3(Vq MPM) -> MPM_Vq/1

== system ThreePhaseVectorControl/Vector Current Controller + PWM/MPM theta ==
  1 : Inport
  2 : Inport  Port=2
  3 : Inport  Port=3
  " 1 " : DataTypeConversion  SaturateOnIntegerOverflow=on  RndMeth=Zero
  " 2 " : DataTypeConversion  SaturateOnIntegerOverflow=on  RndMeth=Zero
  " 3 " : DataTypeConversion  SaturateOnIntegerOverflow=on  RndMeth=Zero
  " InputMux " : Mux  Inputs=3
  " S-Function " : S-Function  FunctionName=plecs  SFunctionDeploymentMode=off  EnableBusSupport=off
  wires:
  " InputMux "/1 -> " S-Function "/1
  1/1 -> " 1 "/1
  " 1 "/1 -> " InputMux "/1
  2/1 -> " 2 "/1
  " 2 "/1 -> " InputMux "/2
  3/1 -> " 3 "/1
  " 3 "/1 -> " InputMux "/3

== system ThreePhaseVectorControl/Vector Current Controller + PWM/MPM//SRF CF ==
  Vabc : Inport
  vg_a : Inport  Port=2
  2*pi3 : Step  Time=0  After=2*pi  SampleTime=0
  Add : Sum
  Clock1 : Clock
      settings: Decimation=100
  Constant7 : Constant  Value=50
  Constant8 : Constant  Value=2*pi
  Gain : Gain  Gain=0.05
  Gain1 : Gain  Gain=0.95
  Integrator3 : Integrator  InitialCondition=0.000000001  UpperSaturationLimit=2*pi  LowerSaturationLimit=0  IgnoreLimit=on
  MPM : Subsystem
  MPM (forcing Vq=0) : Subsystem
  Math Function3 : Math  Operator=mod  SignedPower=on  SaturateOnIntegerOverflow=on
  Product3 : Product  RndMeth=Zero
  SRF_PLL : Subsystem
  Switch1 : Switch  Criteria=u2 > Threshold  Threshold=0.1
  Transfer Fcn1 : TransferFcn  Denominator=[1/(2*pi*100) 1]
  CF_theta : Outport
  CF_Vd : Outport  Port=2
  CF_Vq : Outport  Port=3
  CF_freq : Outport  Port=4
  wires:
  vg_a/1 -> MPM/1(v_g)
  MPM (forcing Vq=0)/1(CF_theta) -> CF_theta/1
  MPM (forcing Vq=0)/2(Vd CF) -> CF_Vd/1
  MPM (forcing Vq=0)/3(Vq CF) -> CF_Vq/1
  Integrator3/1 -> Math Function3/1
  Product3/1 -> Integrator3/1
  2*pi3/1 -> Product3/2
  Math Function3/1 -> MPM (forcing Vq=0)/2(CF theta)
  Constant8/1 -> Math Function3/2
  Vabc/1 -> MPM (forcing Vq=0)/1(Vabc-PLL), SRF_PLL/1(Vabc-PLL)
  Add/1 -> CF_freq/1, Product3/1
  Gain/1 -> Add/1
  Gain1/1 -> Add/2
  MPM/1(MPM freq) -> Gain/1
  Clock1/1 -> Switch1/2
  Constant7/1 -> Switch1/3
  SRF_PLL/1(SRF_freq) -> Switch1/1
  Switch1/1 -> Transfer Fcn1/1
  Transfer Fcn1/1 -> Gain1/1

== system ThreePhaseVectorControl/Vector Current Controller + PWM/PQ ==
  1 : Inport
  2 : Inport  Port=2
  " 1 " : DataTypeConversion  SaturateOnIntegerOverflow=on  RndMeth=Zero
  " 2 " : DataTypeConversion  SaturateOnIntegerOverflow=on  RndMeth=Zero
  " InputMux " : Mux  Inputs=2
  " S-Function " : S-Function  FunctionName=plecs  SFunctionDeploymentMode=off  EnableBusSupport=off
  wires:
  " InputMux "/1 -> " S-Function "/1
  1/1 -> " 1 "/1
  " 1 "/1 -> " InputMux "/1
  2/1 -> " 2 "/1
  " 2 "/1 -> " InputMux "/2

== system ThreePhaseVectorControl/Vector Current Controller + PWM/PWM ==
  Vtabc : Inport
  " tri_sin" : Scope
  Demux1 : Demux  Outputs=3
  Divide : Product  Inputs=/*
  Logical Operator : Logic  Operator=NOT  AllPortsSameDT=off  OutDataTypeStr=boolean
  Logical Operator1 : Logic  Operator=NOT  AllPortsSameDT=off  OutDataTypeStr=boolean
  Logical Operator2 : Logic  Operator=NOT  AllPortsSameDT=off  OutDataTypeStr=boolean
  Mux : Mux
  Relational Operator : RelationalOperator  Operator=<=  OutDataTypeStr=boolean  ZeroCross=off  RndMeth=Nearest
  Relational Operator1 : RelationalOperator  Operator=<=  OutDataTypeStr=boolean  ZeroCross=off  RndMeth=Nearest
  Relational Operator2 : RelationalOperator  Operator=<=  OutDataTypeStr=boolean  ZeroCross=off  RndMeth=Nearest
  Triangle Generator1 : powerlib_meascontrol/Pulse & Signal Generators/Triangle Generator  Freq=5000  Phase=90  Ts=0
  Vdc/2 : Constant  Value=Vdc/2
  gpa : Outport  VectorParamsAs1DForOutWhenUnconnected=off
  gna : Outport  Port=2  VectorParamsAs1DForOutWhenUnconnected=off
  gpb : Outport  Port=3  VectorParamsAs1DForOutWhenUnconnected=off
  gnb : Outport  Port=4  VectorParamsAs1DForOutWhenUnconnected=off
  gpc : Outport  Port=5  VectorParamsAs1DForOutWhenUnconnected=off
  gnc : Outport  Port=6  VectorParamsAs1DForOutWhenUnconnected=off
  PWM trig sin : Outport  Port=7
  wires:
  Triangle Generator1/1 -> Mux/1, Relational Operator/1, Relational Operator1/1, Relational Operator2/1
  Relational Operator/1 -> Logical Operator/1, gpa/1
  Relational Operator1/1 -> Logical Operator1/1, gpb/1
  Relational Operator2/1 -> Logical Operator2/1, gpc/1
  Mux/1 -> " tri_sin"/1, PWM trig sin/1
  Vdc/2/1 -> Divide/1
  Divide/1 -> Demux1/1
  Demux1/1 -> Relational Operator/2, Mux/2
  Demux1/2 -> Relational Operator1/2, Mux/3
  Demux1/3 -> Relational Operator2/2, Mux/4
  Logical Operator/1 -> gna/1
  Vtabc/1 -> Divide/2
  Logical Operator1/1 -> gnb/1
  Logical Operator2/1 -> gnc/1

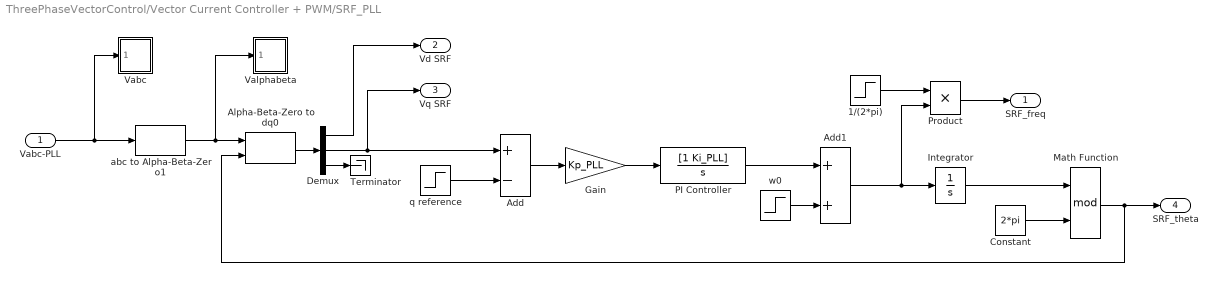
== system ThreePhaseVectorControl/Vector Current Controller + PWM/SRF_PLL ==
  Vabc-PLL : Inport
  1/(2*pi) : Step  Time=0  After=1/(2*pi)  SampleTime=0
  Add : Sum  Inputs=+-
  Add1 : Sum
  Alpha-Beta-Zero to dq0 : powerlib_meascontrol/Transformations/Alpha-Beta-Zero to dq0  Alignment=Aligned with phase A axis
  Constant : Constant  Value=2*pi
  Demux : Demux  Outputs=3
  Gain : Gain  Gain=Kp_PLL
  Integrator : Integrator  UpperSaturationLimit=2*pi  LowerSaturationLimit=0  IgnoreLimit=on
  Math Function : Math  Operator=mod  SignedPower=on  SaturateOnIntegerOverflow=on
  PI Controller : TransferFcn  Numerator=[1 Ki_PLL]  Denominator=[1 0]
  Product : Product  RndMeth=Zero
  Terminator : Terminator
  Vabc : Subsystem  LoadFcn=plecs('sl', 300);  InitFcn=plecs('sl', 314);  StartFcn=plecs('sl', 308);  StopFcn=plecs('sl', 309);  mask{Settings=<binary blob, 1052 chars, not shown>}
      mask init:
      | plecs('sl', 315);
      settings: CopyFcn=plecs('sl', 303);  DeleteFcn=plecs('sl', 305);  UndoDeleteFcn=plecs('sl', 306);  PreSaveFcn=plecs('sl', 311);  NameChangeFcn=plecs('sl', 310);  DestroyFcn=plecs('sl', 307);  OpenFcn=plecs('sl', 302);  ErrorFcn=plerrorfcn
      mask Display: plot([0.1 0.9 0.9 0.1 0.1], [0.9 0.9 0.5 0.5 0.9])
  Valphabeta : Subsystem  LoadFcn=plecs('sl', 300);  InitFcn=plecs('sl', 314);  StartFcn=plecs('sl', 308);  StopFcn=plecs('sl', 309);  mask{Settings=<binary blob, 236 chars, not shown>}
      mask init:
      | plecs('sl', 315);
      settings: CopyFcn=plecs('sl', 303);  DeleteFcn=plecs('sl', 305);  UndoDeleteFcn=plecs('sl', 306);  PreSaveFcn=plecs('sl', 311);  NameChangeFcn=plecs('sl', 310);  DestroyFcn=plecs('sl', 307);  OpenFcn=plecs('sl', 302);  ErrorFcn=plerrorfcn
      mask Display: plot([0.1 0.9 0.9 0.1 0.1], [0.9 0.9 0.5 0.5 0.9])
  abc to Alpha-Beta-Zero1 : powerlib_meascontrol/Transformations/abc to Alpha-Beta-Zero
  q reference : Step  Time=0  After=0  SampleTime=0
  w0 : Step  Time=0  After=2*pi*50  SampleTime=0
  SRF_freq : Outport
  Vd SRF : Outport  Port=2  VectorParamsAs1DForOutWhenUnconnected=off
  Vq SRF : Outport  Port=3  VectorParamsAs1DForOutWhenUnconnected=off
  SRF_theta : Outport  Port=4
  wires:
  Add1/1 -> Product/2, Integrator/1
  Alpha-Beta-Zero to dq0/1 -> Demux/1
  Constant/1 -> Math Function/2
  Demux/3 -> Terminator/1
  1/(2*pi)/1 -> Product/1
  q reference/1 -> Add/2
  Integrator/1 -> Math Function/1
  Product/1 -> SRF_freq/1
  Add/1 -> Gain/1
  Gain/1 -> PI Controller/1
  w0/1 -> Add1/2
  PI Controller/1 -> Add1/1
  abc to Alpha-Beta-Zero1/1 -> Valphabeta/1(1), Alpha-Beta-Zero to dq0/1
  Math Function/1 -> SRF_theta/1, Alpha-Beta-Zero to dq0/2
  Demux/1 -> Vd SRF/1
  Demux/2 -> Vq SRF/1, Add/1
  Vabc-PLL/1 -> Vabc/1(1), abc to Alpha-Beta-Zero1/1

== system ThreePhaseVectorControl/Vector Current Controller + PWM/Scope1 ==
  1 : Inport
  " InputMux " : Subsystem
      mask Display: disp('Mux')
  " S-Function " : S-Function  FunctionName=plecs  SFunctionDeploymentMode=off  EnableBusSupport=off
  wires:
  1/1 -> " InputMux "/1(In1)
  " InputMux "/1(Out) -> " S-Function "/1

== system ThreePhaseVectorControl/Vector Current Controller + PWM/Standard CF ==
  Sensor 1 : Inport
  Sensor 2 : Inport  Port=2
  Add : Sum
  G1 : TransferFcn  Numerator=[2*wc wc^2]  Denominator=[1 2*wc wc^2]
  G2 : TransferFcn  Numerator=[1 0 0]  Denominator=[1 2*wc wc^2]
  CF_freq : Outport
  wires:
  Add/1 -> CF_freq/1
  Sensor 1/1 -> G1/1
  G1/1 -> Add/1
  G2/1 -> Add/2
  Sensor 2/1 -> G2/1

== system ThreePhaseVectorControl/Vector Current Controller + PWM/Three signals CF ==
  Sensor 1 : Inport
  Sensor 2 : Inport  Port=2
  Sensor 3 : Inport  Port=3
  1-G1-G2 : TransferFcn  Numerator=[1 0 ]  Denominator=[1 wc2]
  Add : Sum  Inputs=+++
  G1 : TransferFcn  Denominator=[(1/wc1) 1]
  G2 : TransferFcn  Numerator=[(wb/Q) 0]  Denominator=[1 (wb/Q) wb^2]
  CF_freq : Outport
  wires:
  Add/1 -> CF_freq/1
  G1/1 -> Add/1
  G2/1 -> Add/2
  1-G1-G2/1 -> Add/3
  Sensor 2/1 -> G2/1
  Sensor 3/1 -> 1-G1-G2/1
  Sensor 1/1 -> G1/1

== system ThreePhaseVectorControl/Vector Current Controller + PWM/Vabc & Iabc ==
  1 : Inport
  2 : Inport  Port=2
  " 1 " : DataTypeConversion  SaturateOnIntegerOverflow=on  RndMeth=Zero
  " 2 " : DataTypeConversion  SaturateOnIntegerOverflow=on  RndMeth=Zero
  " InputMux " : Mux  Inputs=2
  " S-Function " : S-Function  FunctionName=plecs  SFunctionDeploymentMode=off  EnableBusSupport=off
  wires:
  " InputMux "/1 -> " S-Function "/1
  1/1 -> " 1 "/1
  " 1 "/1 -> " InputMux "/1
  2/1 -> " 2 "/1
  " 2 "/1 -> " InputMux "/2

== system ThreePhaseVectorControl/Vector Current Controller + PWM/i_dq ==
  1 : Inport
  2 : Inport  Port=2
  " 1 " : DataTypeConversion  SaturateOnIntegerOverflow=on  RndMeth=Zero
  " 2 " : DataTypeConversion  SaturateOnIntegerOverflow=on  RndMeth=Zero
  " InputMux " : Mux  Inputs=2
  " S-Function " : S-Function  FunctionName=plecs  SFunctionDeploymentMode=off  EnableBusSupport=off
  wires:
  " InputMux "/1 -> " S-Function "/1
  1/1 -> " 1 "/1
  " 1 "/1 -> " InputMux "/1
  2/1 -> " 2 "/1
  " 2 "/1 -> " InputMux "/2

== system ThreePhaseVectorControl/Vector Current Controller + PWM/v_dq ==
  1 : Inport
  2 : Inport  Port=2
  " 1 " : DataTypeConversion  SaturateOnIntegerOverflow=on  RndMeth=Zero
  " 2 " : DataTypeConversion  SaturateOnIntegerOverflow=on  RndMeth=Zero
  " InputMux " : Mux  Inputs=2
  " S-Function " : S-Function  FunctionName=plecs  SFunctionDeploymentMode=off  EnableBusSupport=off
  wires:
  " InputMux "/1 -> " S-Function "/1
  1/1 -> " 1 "/1
  " 1 "/1 -> " InputMux "/1
  2/1 -> " 2 "/1
  " 2 "/1 -> " InputMux "/2

== system ThreePhaseVectorControl/Vector Current Controller + PWM/CF/MPM ==
  va : Inport
  Buffer : Buffer  N=500  V=499  ic=zeros(500,1)  OutputFrames=off
  Clock3 : Clock
      settings: Decimation=100
  Constant : Constant  Value=250
  Constant1 : Constant  Value=50
  Constant2 : Constant  Value=MPM_Ts
  Constant4 : Constant  Value=50
  MPM method : MATLAB Function  TreatAsAtomicUnit=on
  Switch3 : Switch  Criteria=u2 > Threshold  Threshold=0.1
  Zero-Order Hold : ZeroOrderHold  SampleTime=MPM_Ts
  MPM freq : Outport
  wires:
  Constant/1 -> MPM method/2(L)
  Zero-Order Hold/1 -> Buffer/1
  Constant1/1 -> MPM method/4(freq_guess)
  Buffer/1 -> MPM method/1(x)
  Clock3/1 -> Switch3/2
  Constant4/1 -> Switch3/3
  Constant2/1 -> MPM method/3(timestep)
  MPM method/1(outputfreq) -> Switch3/1
  va/1 -> Zero-Order Hold/1
  Switch3/1 -> MPM freq/1

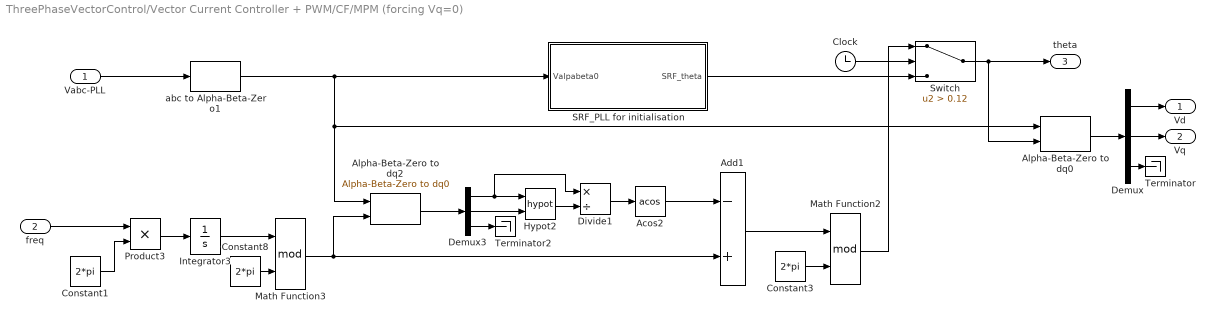
== system ThreePhaseVectorControl/Vector Current Controller + PWM/CF/MPM (forcing Vq=0) ==
  Vabc-PLL : Inport
  freq : Inport  Port=2
  Acos2 : Trigonometry  Operator=acos
  Add1 : Sum  Inputs=-+
  Alpha-Beta-Zero to dq0 : powerlib_meascontrol/Transformations/Alpha-Beta-Zero to dq0  Alignment=Aligned with phase A axis
  Alpha-Beta-Zero to dq2 : powerlib_meascontrol/Transformations/Alpha-Beta-Zero to dq0  Alignment=Aligned with phase A axis
  Clock : Clock
  Constant1 : Constant  Value=2*pi
  Constant3 : Constant  Value=2*pi
  Constant8 : Constant  Value=2*pi
  Demux : Demux  Outputs=3
  Demux3 : Demux  Outputs=3
  Divide1 : Product  Inputs=*/
  Hypot2 : Math  Operator=hypot  SaturateOnIntegerOverflow=on
  Integrator3 : Integrator  UpperSaturationLimit=2*pi  LowerSaturationLimit=0  IgnoreLimit=on
  Math Function2 : Math  Operator=mod  SignedPower=on  SaturateOnIntegerOverflow=on
  Math Function3 : Math  Operator=mod  SignedPower=on  SaturateOnIntegerOverflow=on
  Product3 : Product  RndMeth=Zero
  SRF_PLL for initialisation : Subsystem
  Switch : Switch  Criteria=u2 > Threshold  Threshold=0.12
  Terminator : Terminator
  Terminator2 : Terminator
  abc to Alpha-Beta-Zero1 : powerlib_meascontrol/Transformations/abc to Alpha-Beta-Zero
  Vd : Outport
  Vq : Outport  Port=2
  theta : Outport  Port=3  VectorParamsAs1DForOutWhenUnconnected=off
  wires:
  Add1/1 -> Math Function2/1
  Alpha-Beta-Zero to dq2/1 -> Demux3/1
  Demux3/3 -> Terminator2/1
  Constant3/1 -> Math Function2/2
  Math Function2/1 -> Switch/1
  Clock/1 -> Switch/2
  SRF_PLL for initialisation/1(SRF_theta) -> Switch/3
  Switch/1 -> theta/1, Alpha-Beta-Zero to dq0/2
  Divide1/1 -> Acos2/1
  Hypot2/1 -> Divide1/2
  Acos2/1 -> Add1/1
  Demux3/1 -> Hypot2/1, Divide1/1
  Demux3/2 -> Hypot2/2
  Vabc-PLL/1 -> abc to Alpha-Beta-Zero1/1
  Integrator3/1 -> Math Function3/1
  Constant1/1 -> Product3/2
  Product3/1 -> Integrator3/1
  Constant8/1 -> Math Function3/2
  freq/1 -> Product3/1
  Math Function3/1 -> Alpha-Beta-Zero to dq2/2, Add1/2
  abc to Alpha-Beta-Zero1/1 -> SRF_PLL for initialisation/1(Valpabeta0), Alpha-Beta-Zero to dq0/1, Alpha-Beta-Zero to dq2/1
  Alpha-Beta-Zero to dq0/1 -> Demux/1
  Demux/3 -> Terminator/1
  Demux/2 -> Vq/1
  Demux/1 -> Vd/1

== system ThreePhaseVectorControl/Vector Current Controller + PWM/CF/SRF PLL ==
  Vabc : Inport
  1/(2*pi) : Step  Time=0  After=1/(2*pi)  SampleTime=0
  Add : Sum  Inputs=+-
  Add1 : Sum
  Constant : Constant  Value=2*pi
  Demux : Demux  Outputs=3
  Gain : Gain  Gain=Kp_PLL
  Integrator : Integrator  UpperSaturationLimit=2*pi  LowerSaturationLimit=0  IgnoreLimit=on
  Math Function : Math  Operator=mod  SignedPower=on  SaturateOnIntegerOverflow=on
  PI Controller : TransferFcn  Numerator=[1 Ki_PLL]  Denominator=[1 0]
  Product : Product  RndMeth=Zero
  Terminator : Terminator
  Terminator1 : Terminator
  abc to dq0 : powerlib_meascontrol/Transformations/abc to dq0  Alignment=Aligned with phase A axis
  q reference : Step  Time=0  After=0  SampleTime=0
  w0 : Step  Time=0  After=2*pi*50  SampleTime=0
  frequency : Outport
  delta_w0 : Outport  Port=2
  wires:
  Vabc/1 -> abc to dq0/1
  Integrator/1 -> Math Function/1
  Gain/1 -> PI Controller/1
  Add1/1 -> Product/2, Integrator/1
  Demux/2 -> Add/1
  w0/1 -> Add1/2
  q reference/1 -> Add/2
  1/(2*pi)/1 -> Product/1
  Product/1 -> frequency/1
  PI Controller/1 -> Add1/1, delta_w0/1
  Constant/1 -> Math Function/2
  Demux/3 -> Terminator/1
  Add/1 -> Gain/1
  abc to dq0/1 -> Demux/1
  Math Function/1 -> abc to dq0/2
  Demux/1 -> Terminator1/1
